simulink model "FOC_CHBI"  (R2025a)
settings: Solver=VariableStepAuto  StartTime=0.0  StopTime=6.5  RelTol=1e-3
InitFcn:
  | %% KHOI THONG SO DONG CO
  | U_nom=6000;%6600;           %dien ap dinh muc dong co
  | H=0.96;%0.9387;             %hieu suat dong co
  | Pn=1e6;%1750e3;         %Cong suat dinh muc dong co
  | cosphi=0.85;%0.9297;        %He so cong suat
  | Sn=Pn/cosphi;       %Cong suat toan phan
  | J=27.9;%34.8;                %Moment quan tinh
  | pc=2;%2;               %So cap cuc
  | fn=50;              %Tan so luoi
  | n=1490;%1486;             %Toc do dinh muc 2880
  | Mdm=6153;%(9.55*Pn*H)/n;  %Moment dinh muc
  | In=117;%Pn/(U_nom*H*cosphi*sqrt(3))   ;
  | Isd=sqrt(2)*In*sqrt(1-cosphi);
  | Isq=sqrt(2*In^2-Isd^2);
  | wrn=2*pi*(fn-(pc*n/60));               %Toc do truotdinh muc
  | Tr=Isq/(wrn*Isd) ;                   %Tinh 'Tr'trong cac cong thuc
  | %Xo=(sqrt(1-cosphi^2)-cosphi*Isd/Isq)*(Un*sqrt(2)/(sqrt(3)*In));
  | Xo=(sqrt(1-cosphi^2)-cosphi*Isd/Isq)*(U_nom/(sqrt(3)*In));
  | Xh=sqrt(2/3)*(U_nom/Isd) - Xo;
  | Rs=(wrn*Isd*Xh)/(2*pi*fn*Isq);
  | Rr=Rs;
  | o=Xo/Xh;
  | Ts=Xh/(2*pi*fn*Rs);
  | Tos=o*Ts;
  | Lr=Tr*Rr;
  | Lor=o*Lr;
  | Ls=Ts*Rs;
  | Los=o*Ls;
  | Lm=sqrt((1-o)*Ls*Lr);
  | %tham so dong co 2850e3Kw
  | %Rs=0.05;
  | %Rr = 0.062;
  | %Los = 0.957/(100*pi);
  | %Lor = 2.237/(100*pi);
  | %Lm = 34.826/(100*pi);
  | %Ts = (Lm +Los)/Rs;
  | %Tr = (Lm+Lor)/Rr;
  | %Lr = Lm + Lor;
  | %Ls = Lm + Los;
  | Udc = 1.1*6000/(0.612*12);%6600/(0.612*12);
  | Rt =18*Udc*Udc/1e6; %18*Udc*Udc/2010.6e3;
  | C_f = 5/(6*100*pi*Rt*0.001);
  | %Fan and Pumb Load Coeficient
  | TL0 = (2.0/100)*Mdm; %(2.0/100)*TN;
  | Omega_rated = n/9.55; %nN/9.55; %rad/s
  | LoadGain = (Mdm - TL0)/(Omega_rated*Omega_rated);
  | fs=5000;
  | %% THAM SO CAC BO DIEU KHIEN
  | %---------------- control volocity
  | epxilon = 0.7;
  | wn = 40;
  |      %P_w = (2*epxilon*wn*J)/pc;
  |     %I_w = wn*wn*J/pc;
  |  P_w = 60;%5;%15;%9;%12;%10;%(2*epxilon*wn*J)/pc
  |  I_w = 80;%150;%80;%100;%40;%50;%wn*wn*J/pc
  | %---------------- control current
  |     %P_id = Rs*Tos*fs/5;
  |     % I_id = Rs*Tos*fs/5/Tos;
  |      %P_iq = P_id;
  |      %I_iq = I_id;
  | ... (+9 lines)
StopFcn:
  | figure(1);
  | subplot(1,1,1); hold on; grid on;
  | plot(phi_ref.time, phi_ref.signals.values,'r--', 'Linewidth',1.5);
  | plot(phi.time, phi.signals.values,'b', 'Linewidth',1.5);
  | legend('phi*-rd','phi-rd');
  | title('Từ thông');
  | xlabel('Thời gian (s)'); ylabel('Wb');
  | 
  | 
  | figure(2);
  | subplot(2,1,1); hold on; grid on;
  | plot(torque.time, torque.signals.values,'r','Linewidth',1.5);
  | legend('Te');
  | title('Mô-men');
  | xlabel('Thời gian (s)'); ylabel('Nm');
  | 
  | subplot(2,1,2); hold on; grid on;
  | plot(speed_ref.time, speed_ref.signals.values,'r--','Linewidth',1.5);
  | plot(speed.time, speed.signals.values,'b','Linewidth',1.5);
  | legend('Tốc độ đặt','Tốc độ thực');
  | title('Tốc độ');
  | xlabel('Thời gian (s)'); ylabel('RPM');
  | 
  | figure(3)
  | 
  | subplot(2,1,1); hold on; grid on;
  | plot(isd_ref.time, isd_ref.signals.values,'r','Linewidth',1.5);
  | plot(isd.time, isd.signals.values,'b','Linewidth',1.5);
  | legend('isd*','isd');
  | title('Dòng điện isd');
  | xlabel('Thời gian (s)'); ylabel('A');
  | 
  | subplot(2,1,2); hold on; grid on;
  | plot(isq_ref.time, isq_ref.signals.values,'r','Linewidth',1.5);
  | plot(isq.time, isq.signals.values,'b','Linewidth',1.5);
  | legend('isq*','isq');
  | title('Dòng điện isq');
  | xlabel('Thời gian (s)'); ylabel('A');
  | 
  | figure(4)
  | 
  | subplot(2,1,1); hold on; grid on;
  | plot(va.time, va.signals.values,'b','Linewidth',1.5);
  | plot(vb.time, vb.signals.values,'k','Linewidth',1.5);
  | plot(vc.time, vc.signals.values,'r','Linewidth',1.5);
  | legend('Ua','Ub','Uc');
  | title('Điện áp pha');
  | xlabel('Thời gian (s)'); ylabel('V');
  | 
  | subplot(2,1,2); hold on; grid on;
  | plot(vab.time, vab.signals.values,'k','Linewidth',1.5);
  | plot(vbc.time, vbc.signals.values,'b','Linewidth',1.5);
  | plot(vca.time, vca.signals.values,'r','Linewidth',1.5);
  | legend('Uab','Ubc','Uca');
  | title('Điện áp dây');
  | xlabel('Thời gian (s)'); ylabel('V');
  | 
  | figure(5);
  | subplot(1,1,1); hold on; grid on;
  | plot(Ia.time, Ia.signals.values,'k','Linewidth',1.5);
  | ... (+5 lines)
undefined symbols (not defined in the file): sigbuilder_block
libraries: spsIGBTDiodeLib x72, spsTriangleGeneratorLib x36, spsSeriesRLCBranchLib x18, spsBreakerLib x18, spsUniversalBridgeLib x18, spsZigzagPhaseShiftingTransformerLib x15, spsVoltageMeasurementLib x8, spsACVoltageSourceLib x3, spsCurrentMeasurementLib x3, spsThreePhaseTransformerTwoWindingsLib x3, slpidlib x2, spsThreePhaseVIMeasurementLib x1
(part 3 of 3)

== system FOC_CHBI/CASECADED H-BRIDGE INVERTER/POWER CIRCUIT1/Subsystem1/Subsystem4 ==
  PWM : Inport
  Breaker : spsBreakerLib/Breaker  InitialState=0  SwitchingTimes="[1/60  5/60]"  External=on  BreakerResistance=0.01  SnubberResistance=1e6  SnubberCapacitance=inf  Measurements=None  MoreParameters=on  NoBreakLoop=off
  Demux : Demux  Outputs=2
  IGBT/Diode{1..4} (4 alike) : spsIGBTDiodeLib/IGBT//Diode  Ron=1e-3  Rs=1e5  Cs=inf  Measurements=off
  Logical Operator : Logic  Operator=NOT  AllPortsSameDT=off  OutDataTypeStr=boolean
  Logical Operator1 : Logic  Operator=NOT  AllPortsSameDT=off  OutDataTypeStr=boolean
  Step : Step  Time=0  After=0  SampleTime=0
  A : PMIOPort  Side=Right
  B : PMIOPort  Port=2  Side=Right
  + : PMIOPort  Port=3  Side=Left
  - : PMIOPort  Port=4  Side=Left
  tag scope: eCH4=global
  wires:
  Step/1 -> Breaker/1, [eCH4]
  Logical Operator1/1 -> IGBT/Diode2/1
  Demux/2 -> Logical Operator1/1, IGBT/Diode3/1
  Logical Operator/1 -> IGBT/Diode4/1
  Demux/1 -> Logical Operator/1, IGBT/Diode1/1
  PWM/1 -> Demux/1
  connections:
  IGBT/Diode4/RConn1 -- -/RConn1 -- IGBT/Diode2/RConn1
  IGBT/Diode3/RConn1 -- B/RConn1 -- Breaker/RConn1 -- IGBT/Diode2/LConn1
  IGBT/Diode4/LConn1 -- A/RConn1 -- Breaker/LConn1 -- IGBT/Diode1/RConn1
  IGBT/Diode3/LConn1 -- +/RConn1 -- IGBT/Diode1/LConn1

== system FOC_CHBI/CASECADED H-BRIDGE INVERTER/POWER CIRCUIT1/Subsystem1/Subsystem6 ==
  PWM : Inport
  Breaker : spsBreakerLib/Breaker  InitialState=0  SwitchingTimes="[1/60  5/60]"  External=on  BreakerResistance=0.01  SnubberResistance=1e6  SnubberCapacitance=inf  Measurements=None  MoreParameters=on  NoBreakLoop=off
  Constant : Constant  Value=0
  Demux : Demux  Outputs=2
  IGBT/Diode{1..4} (4 alike) : spsIGBTDiodeLib/IGBT//Diode  Ron=1e-3  Rs=1e5  Cs=inf  Measurements=off
  Logical Operator : Logic  Operator=NOT  AllPortsSameDT=off  OutDataTypeStr=boolean
  Logical Operator1 : Logic  Operator=NOT  AllPortsSameDT=off  OutDataTypeStr=boolean
  Step : Step  Time=4  SampleTime=0
  Step1 : Step  Time=4  Before=1  After=-1  SampleTime=0
  Switch{,1..3} (4 alike) : Switch  Criteria=u2 > Threshold  SaturateOnIntegerOverflow=off  InputSameDT=off
  A : PMIOPort  Side=Right
  B : PMIOPort  Port=2  Side=Right
  + : PMIOPort  Port=3  Side=Left
  - : PMIOPort  Port=4  Side=Left
  tag scope: eCH5=global
  wires:
  Demux/2 -> Switch1/1, Logical Operator1/1
  Logical Operator/1 -> Switch2/3, Switch2/1
  Demux/1 -> Switch/1, Logical Operator/1
  PWM/1 -> Demux/1
  Step/1 -> [eCH5], Breaker/1
  Switch/1 -> IGBT/Diode1/1
  Switch1/1 -> IGBT/Diode3/1
  Switch2/1 -> IGBT/Diode4/1
  Logical Operator1/1 -> Switch3/1
  Switch3/1 -> IGBT/Diode2/1
  Constant/1 -> Switch/3, Switch1/3, Switch3/3
  Step1/1 -> Switch2/2, Switch3/2, Switch1/2, Switch/2
  connections:
  IGBT/Diode4/RConn1 -- -/RConn1 -- IGBT/Diode2/RConn1
  IGBT/Diode3/RConn1 -- Breaker/RConn1 -- B/RConn1 -- IGBT/Diode2/LConn1
  IGBT/Diode4/LConn1 -- Breaker/LConn1 -- A/RConn1 -- IGBT/Diode1/RConn1
  IGBT/Diode3/LConn1 -- +/RConn1 -- IGBT/Diode1/LConn1

== system FOC_CHBI/CASECADED H-BRIDGE INVERTER/POWER CIRCUIT1/Subsystem1/Subsystem7 ==
  PWM : Inport
  Breaker : spsBreakerLib/Breaker  InitialState=0  SwitchingTimes="[1/60  5/60]"  External=on  BreakerResistance=0.01  SnubberResistance=1e6  SnubberCapacitance=inf  Measurements=None  MoreParameters=on  NoBreakLoop=off
  Constant : Constant  Value=0
  Demux : Demux  Outputs=2
  IGBT/Diode{1..4} (4 alike) : spsIGBTDiodeLib/IGBT//Diode  Ron=1e-3  Rs=1e5  Cs=inf  Measurements=off
  Logical Operator : Logic  Operator=NOT  AllPortsSameDT=off  OutDataTypeStr=boolean
  Logical Operator1 : Logic  Operator=NOT  AllPortsSameDT=off  OutDataTypeStr=boolean
  Step : Step  Time=4  SampleTime=0
  Step1 : Step  Time=4  Before=1  After=-1  SampleTime=0
  Switch{,1..3} (4 alike) : Switch  Criteria=u2 > Threshold  SaturateOnIntegerOverflow=off  InputSameDT=off
  A : PMIOPort  Side=Right
  B : PMIOPort  Port=2  Side=Right
  + : PMIOPort  Port=3  Side=Left
  - : PMIOPort  Port=4  Side=Left
  tag scope: eCH6=global
  wires:
  Demux/2 -> Switch1/1, Logical Operator1/1
  Logical Operator/1 -> Switch2/3, Switch2/1
  Demux/1 -> Switch/1, Logical Operator/1
  PWM/1 -> Demux/1
  Step/1 -> [eCH6], Breaker/1
  Switch/1 -> IGBT/Diode1/1
  Switch1/1 -> IGBT/Diode3/1
  Switch2/1 -> IGBT/Diode4/1
  Logical Operator1/1 -> Switch3/1
  Switch3/1 -> IGBT/Diode2/1
  Constant/1 -> Switch/3, Switch1/3, Switch3/3
  Step1/1 -> Switch2/2, Switch3/2, Switch1/2, Switch/2
  connections:
  IGBT/Diode4/RConn1 -- -/RConn1 -- IGBT/Diode2/RConn1
  IGBT/Diode3/RConn1 -- Breaker/RConn1 -- B/RConn1 -- IGBT/Diode2/LConn1
  IGBT/Diode4/LConn1 -- Breaker/LConn1 -- A/RConn1 -- IGBT/Diode1/RConn1
  IGBT/Diode3/LConn1 -- +/RConn1 -- IGBT/Diode1/LConn1

== system FOC_CHBI/CASECADED H-BRIDGE INVERTER/POWER CIRCUIT1/Subsystem2/Subsystem1 ==
  PWM : Inport
  Breaker : spsBreakerLib/Breaker  InitialState=0  SwitchingTimes="[1/60  5/60]"  External=on  BreakerResistance=0.01  SnubberResistance=1e6  SnubberCapacitance=inf  Measurements=None  MoreParameters=on  NoBreakLoop=off
  Demux : Demux  Outputs=2
  IGBT/Diode{1..4} (4 alike) : spsIGBTDiodeLib/IGBT//Diode  Ron=1e-3  Rs=1e5  Cs=inf  Measurements=off
  Logical Operator : Logic  Operator=NOT  AllPortsSameDT=off  OutDataTypeStr=boolean
  Logical Operator1 : Logic  Operator=NOT  AllPortsSameDT=off  OutDataTypeStr=boolean
  Step : Step  Time=0  After=0  SampleTime=0
  A : PMIOPort  Side=Right
  B : PMIOPort  Port=2  Side=Right
  + : PMIOPort  Port=3  Side=Left
  - : PMIOPort  Port=4  Side=Left
  tag scope: eAH1=global
  wires:
  Step/1 -> Breaker/1, [eAH1]
  Demux/1 -> Logical Operator/1, IGBT/Diode1/1
  PWM/1 -> Demux/1
  Logical Operator/1 -> IGBT/Diode4/1
  Demux/2 -> IGBT/Diode3/1, Logical Operator1/1
  Logical Operator1/1 -> IGBT/Diode2/1
  connections:
  IGBT/Diode1/LConn1 -- +/RConn1 -- IGBT/Diode3/LConn1
  IGBT/Diode1/RConn1 -- A/RConn1 -- Breaker/LConn1 -- IGBT/Diode4/LConn1
  IGBT/Diode2/LConn1 -- B/RConn1 -- Breaker/RConn1 -- IGBT/Diode3/RConn1
  IGBT/Diode2/RConn1 -- -/RConn1 -- IGBT/Diode4/RConn1

== system FOC_CHBI/CASECADED H-BRIDGE INVERTER/POWER CIRCUIT1/Subsystem2/Subsystem2 ==
  PWM : Inport
  Breaker : spsBreakerLib/Breaker  InitialState=0  SwitchingTimes="[1/60  5/60]"  External=on  BreakerResistance=0.01  SnubberResistance=1e6  SnubberCapacitance=inf  Measurements=None  MoreParameters=on  NoBreakLoop=off
  Demux : Demux  Outputs=2
  IGBT/Diode{1..4} (4 alike) : spsIGBTDiodeLib/IGBT//Diode  Ron=1e-3  Rs=1e5  Cs=inf  Measurements=off
  Logical Operator : Logic  Operator=NOT  AllPortsSameDT=off  OutDataTypeStr=boolean
  Logical Operator1 : Logic  Operator=NOT  AllPortsSameDT=off  OutDataTypeStr=boolean
  Step : Step  Time=0  After=0  SampleTime=0
  A : PMIOPort  Side=Right
  B : PMIOPort  Port=2  Side=Right
  + : PMIOPort  Port=3  Side=Left
  - : PMIOPort  Port=4  Side=Left
  tag scope: eAH2=global
  wires:
  Step/1 -> Breaker/1, [eAH2]
  Logical Operator1/1 -> IGBT/Diode2/1
  Demux/2 -> Logical Operator1/1, IGBT/Diode3/1
  Logical Operator/1 -> IGBT/Diode4/1
  Demux/1 -> Logical Operator/1, IGBT/Diode1/1
  PWM/1 -> Demux/1
  connections:
  IGBT/Diode4/RConn1 -- -/RConn1 -- IGBT/Diode2/RConn1
  IGBT/Diode3/RConn1 -- B/RConn1 -- Breaker/RConn1 -- IGBT/Diode2/LConn1
  IGBT/Diode4/LConn1 -- A/RConn1 -- Breaker/LConn1 -- IGBT/Diode1/RConn1
  IGBT/Diode3/LConn1 -- +/RConn1 -- IGBT/Diode1/LConn1

== system FOC_CHBI/CASECADED H-BRIDGE INVERTER/POWER CIRCUIT1/Subsystem2/Subsystem3 ==
  PWM : Inport
  Breaker : spsBreakerLib/Breaker  InitialState=0  SwitchingTimes="[1/60  5/60]"  External=on  BreakerResistance=0.01  SnubberResistance=1e6  SnubberCapacitance=inf  Measurements=None  MoreParameters=on  NoBreakLoop=off
  Demux : Demux  Outputs=2
  IGBT/Diode{1..4} (4 alike) : spsIGBTDiodeLib/IGBT//Diode  Ron=1e-3  Rs=1e5  Cs=inf  Measurements=off
  Logical Operator : Logic  Operator=NOT  AllPortsSameDT=off  OutDataTypeStr=boolean
  Logical Operator1 : Logic  Operator=NOT  AllPortsSameDT=off  OutDataTypeStr=boolean
  Step : Step  Time=0  After=0  SampleTime=0
  A : PMIOPort  Side=Right
  B : PMIOPort  Port=2  Side=Right
  + : PMIOPort  Port=3  Side=Left
  - : PMIOPort  Port=4  Side=Left
  tag scope: eAH3=global
  wires:
  Step/1 -> Breaker/1, [eAH3]
  PWM/1 -> Demux/1
  Demux/1 -> IGBT/Diode1/1, Logical Operator/1
  Logical Operator/1 -> IGBT/Diode4/1
  Demux/2 -> IGBT/Diode3/1, Logical Operator1/1
  Logical Operator1/1 -> IGBT/Diode2/1
  connections:
  IGBT/Diode1/LConn1 -- +/RConn1 -- IGBT/Diode3/LConn1
  IGBT/Diode1/RConn1 -- A/RConn1 -- Breaker/LConn1 -- IGBT/Diode4/LConn1
  IGBT/Diode2/LConn1 -- B/RConn1 -- Breaker/RConn1 -- IGBT/Diode3/RConn1
  IGBT/Diode2/RConn1 -- -/RConn1 -- IGBT/Diode4/RConn1

== system FOC_CHBI/CASECADED H-BRIDGE INVERTER/POWER CIRCUIT1/Subsystem2/Subsystem4 ==
  PWM : Inport
  Breaker : spsBreakerLib/Breaker  InitialState=0  SwitchingTimes="[1/60  5/60]"  External=on  BreakerResistance=0.01  SnubberResistance=1e6  SnubberCapacitance=inf  Measurements=None  MoreParameters=on  NoBreakLoop=off
  Demux : Demux  Outputs=2
  IGBT/Diode{1..4} (4 alike) : spsIGBTDiodeLib/IGBT//Diode  Ron=1e-3  Rs=1e5  Cs=inf  Measurements=off
  Logical Operator : Logic  Operator=NOT  AllPortsSameDT=off  OutDataTypeStr=boolean
  Logical Operator1 : Logic  Operator=NOT  AllPortsSameDT=off  OutDataTypeStr=boolean
  Step : Step  Time=0  After=0  SampleTime=0
  A : PMIOPort  Side=Right
  B : PMIOPort  Port=2  Side=Right
  + : PMIOPort  Port=3  Side=Left
  - : PMIOPort  Port=4  Side=Left
  tag scope: eAH4=global
  wires:
  Step/1 -> Breaker/1, [eAH4]
  Logical Operator1/1 -> IGBT/Diode2/1
  Demux/2 -> Logical Operator1/1, IGBT/Diode3/1
  Logical Operator/1 -> IGBT/Diode4/1
  Demux/1 -> Logical Operator/1, IGBT/Diode1/1
  PWM/1 -> Demux/1
  connections:
  IGBT/Diode4/RConn1 -- -/RConn1 -- IGBT/Diode2/RConn1
  IGBT/Diode3/RConn1 -- B/RConn1 -- Breaker/RConn1 -- IGBT/Diode2/LConn1
  IGBT/Diode4/LConn1 -- A/RConn1 -- Breaker/LConn1 -- IGBT/Diode1/RConn1
  IGBT/Diode3/LConn1 -- +/RConn1 -- IGBT/Diode1/LConn1

== system FOC_CHBI/CASECADED H-BRIDGE INVERTER/POWER CIRCUIT1/Subsystem2/Subsystem5 ==
  PWM : Inport
  Breaker : spsBreakerLib/Breaker  InitialState=0  SwitchingTimes="[1/60  5/60]"  External=on  BreakerResistance=0.01  SnubberResistance=1e6  SnubberCapacitance=inf  Measurements=None  MoreParameters=on  NoBreakLoop=off
  Constant : Constant  Value=0
  Demux : Demux  Outputs=2
  IGBT/Diode{1..4} (4 alike) : spsIGBTDiodeLib/IGBT//Diode  Ron=1e-3  Rs=1e5  Cs=inf  Measurements=off
  Logical Operator : Logic  Operator=NOT  AllPortsSameDT=off  OutDataTypeStr=boolean
  Logical Operator1 : Logic  Operator=NOT  AllPortsSameDT=off  OutDataTypeStr=boolean
  Step : Step  Time=4  SampleTime=0
  Step1 : Step  Time=4  Before=1  After=-1  SampleTime=0
  Switch{,1..3} (4 alike) : Switch  Criteria=u2 > Threshold  SaturateOnIntegerOverflow=off  InputSameDT=off
  A : PMIOPort  Side=Right
  B : PMIOPort  Port=2  Side=Right
  + : PMIOPort  Port=3  Side=Left
  - : PMIOPort  Port=4  Side=Left
  tag scope: eAH5=global
  wires:
  Step1/1 -> Switch/2, Switch1/2, Switch3/2, Switch2/2
  Constant/1 -> Switch3/3, Switch1/3, Switch/3
  Switch3/1 -> IGBT/Diode2/1
  Logical Operator1/1 -> Switch3/1
  Switch2/1 -> IGBT/Diode4/1
  Switch1/1 -> IGBT/Diode3/1
  Switch/1 -> IGBT/Diode1/1
  Step/1 -> Breaker/1, [eAH5]
  PWM/1 -> Demux/1
  Demux/1 -> Logical Operator/1, Switch/1
  Logical Operator/1 -> Switch2/1, Switch2/3
  Demux/2 -> Logical Operator1/1, Switch1/1
  connections:
  IGBT/Diode1/LConn1 -- +/RConn1 -- IGBT/Diode3/LConn1
  IGBT/Diode1/RConn1 -- A/RConn1 -- Breaker/LConn1 -- IGBT/Diode4/LConn1
  IGBT/Diode2/LConn1 -- B/RConn1 -- Breaker/RConn1 -- IGBT/Diode3/RConn1
  IGBT/Diode2/RConn1 -- -/RConn1 -- IGBT/Diode4/RConn1

== system FOC_CHBI/CASECADED H-BRIDGE INVERTER/POWER CIRCUIT1/Subsystem2/Subsystem6 ==
  PWM : Inport
  Breaker : spsBreakerLib/Breaker  InitialState=0  SwitchingTimes="[1/60  5/60]"  External=on  BreakerResistance=0.01  SnubberResistance=1e6  SnubberCapacitance=inf  Measurements=None  MoreParameters=on  NoBreakLoop=off
  Constant : Constant  Value=0
  Demux : Demux  Outputs=2
  IGBT/Diode{1..4} (4 alike) : spsIGBTDiodeLib/IGBT//Diode  Ron=1e-3  Rs=1e5  Cs=inf  Measurements=off
  Logical Operator : Logic  Operator=NOT  AllPortsSameDT=off  OutDataTypeStr=boolean
  Logical Operator1 : Logic  Operator=NOT  AllPortsSameDT=off  OutDataTypeStr=boolean
  Step : Step  Time=4  SampleTime=0
  Step1 : Step  Time=4  Before=1  After=-1  SampleTime=0
  Switch{,1..3} (4 alike) : Switch  Criteria=u2 > Threshold  SaturateOnIntegerOverflow=off  InputSameDT=off
  A : PMIOPort  Side=Right
  B : PMIOPort  Port=2  Side=Right
  + : PMIOPort  Port=3  Side=Left
  - : PMIOPort  Port=4  Side=Left
  tag scope: eAH6=global
  wires:
  Demux/2 -> Switch1/1, Logical Operator1/1
  Logical Operator/1 -> Switch2/3, Switch2/1
  Demux/1 -> Switch/1, Logical Operator/1
  PWM/1 -> Demux/1
  Step/1 -> [eAH6], Breaker/1
  Switch/1 -> IGBT/Diode1/1
  Switch1/1 -> IGBT/Diode3/1
  Switch2/1 -> IGBT/Diode4/1
  Logical Operator1/1 -> Switch3/1
  Switch3/1 -> IGBT/Diode2/1
  Constant/1 -> Switch/3, Switch1/3, Switch3/3
  Step1/1 -> Switch2/2, Switch3/2, Switch1/2, Switch/2
  connections:
  IGBT/Diode4/RConn1 -- -/RConn1 -- IGBT/Diode2/RConn1
  IGBT/Diode3/RConn1 -- Breaker/RConn1 -- B/RConn1 -- IGBT/Diode2/LConn1
  IGBT/Diode4/LConn1 -- Breaker/LConn1 -- A/RConn1 -- IGBT/Diode1/RConn1
  IGBT/Diode3/LConn1 -- +/RConn1 -- IGBT/Diode1/LConn1

== matlab function FOC_CHBI/CASECADED H-BRIDGE INVERTER/CONTROLLER/Giới hạn tốc độ đặt2/MATLAB Function1 ==
  data: Umax input; vt output; e input; v_ref input
function vt = fcn(Umax,e,v_ref)
% dien ap dinh muc cua dong co
%U_nom = 6000;%6600; % voltage
% toc do dinh muc cua dong co
w_nom = 992.263;%1486; % rpm
% toc do cuc dai ung voi dien ap max cua bien tan
%w_max = w_nom*sqrt(Umax/(U_nom*sqrt(2)));% rpm
if e == 0 
    vt = v_ref;
else %e ~0
    if Umax >= 6000*sqrt(2);
        vt = v_ref;
    else %Umax < 690   
        TH = sqrt(Umax/(6000*sqrt(2)))*w_nom;
        if v_ref >= TH
            vt = TH;
        elseif v_ref <= -TH
            vt = -TH;
        else
            vt = v_ref;
        end
    end
end
end

== matlab function FOC_CHBI/CASECADED H-BRIDGE INVERTER/CONTROLLER/R_i1/id/MATLAB Function ==
  data: temp output; uk_1 input; uk output; ek input; ek_1 input; Kp input; Ki input; T input; limit input
function [temp,uk] = PI(uk_1,ek,ek_1,Kp,Ki,T,limit)
temp = uk_1 + ek*(Kp + Ki*T/2) + ek_1*(Ki*T/2 - Kp);
if temp >= limit
    uk = limit;
elseif temp <= -limit
    uk = -limit;
else 
    uk = temp;
end

== matlab function FOC_CHBI/CASECADED H-BRIDGE INVERTER/CONTROLLER/R_i1/iq/MATLAB Function ==
  data: temp output; uk_1 input; uk output; ek input; ek_1 input; Kp input; Ki input; T input; limit input
function [temp,uk] = PI(uk_1,ek,ek_1,Kp,Ki,T,limit)
temp = uk_1 + ek*(Kp + Ki*T/2) + ek_1*(Ki*T/2 - Kp);
if temp >= limit
    uk = limit;
elseif temp <= -limit
    uk = -limit;
else 
    uk = temp;
end
